simulink model "Controlador_com_Observador_Simulink(1)"  (R2019a)
settings: Solver=VariableStepAuto  StartTime=0.0  StopTime=10.0  RelTol=1e-3
values from neighbouring files (symbols this model uses):
  A = [0 1 0;0 0 1;-6 -11 -6]    [Projeto_controlador_observador(2).m]    (also in Q1_PCO(3).m = [0 1; -3 -4]; Q2_PCO(1).m = [0 1 0; 0 0 1; -12 -19 -8]; Q2_PCO(2).m = [0 1 0; 0 0 1; -12 -19 -8]; Q2_PCO(3).m = [0 1 0; 0 0 1; -12 -19 -8])
  B = [0 0 10]'    [Projeto_controlador_observador(2).m]    (also in Q1_PCO(3).m = [0 1]'; Q2_PCO(1).m = [0 0 1]'; Q2_PCO(2).m = [0 0 1]'; Q2_PCO(3).m = [0 0 1]')
  C = [1 0 0]    [Projeto_controlador_observador(2).m]    (also in Q1_PCO(3).m = [3 0]; Q2_PCO(1).m = [2 1 0]; Q2_PCO(2).m = [2 1 0]; Q2_PCO(3).m = [2 1 0])
  Kbar = acker(Abar,Bbar,polosMF)    [Projeto_controlador_observador(2).m]
  Ke = acker(A',C',autovaloresOBSV)'    [Projeto_controlador_observador(2).m]    (also in Q1_PCO(3).m = acker(A', C', autovaloresOBSV)'; Q2_PCO(1).m = acker(A', C', autovaloresOBSV)'; Q2_PCO(2).m = acker(A', C', autovaloresOBSV)'; Q2_PCO(3).m = acker(A', C', autovaloresOBSV)')
settings Model: Creator=rcard  LastModifiedBy=rcard

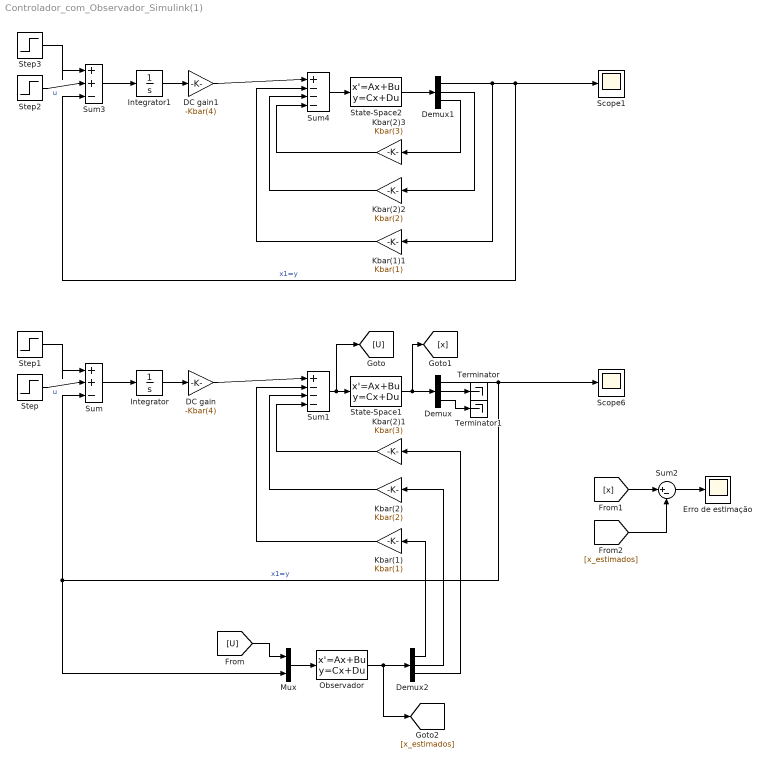
== system Controlador_com_Observador_Simulink(1) ==
  DC gain : Gain  Gain=-Kbar(4)
  DC gain1 : Gain  Gain=-Kbar(4)
  Demux : Demux  Outputs=3
  Demux1 : Demux  Outputs=3
  Demux2 : Demux  Outputs=3
  Erro de estimação : Scope
  Integrator : Integrator
  Integrator1 : Integrator
  Kbar(1) : Gain  Gain=Kbar(1)
  Kbar(1)1 : Gain  Gain=Kbar(1)
  Kbar(2) : Gain  Gain=Kbar(2)
  Kbar(2)1 : Gain  Gain=Kbar(3)
  Kbar(2)2 : Gain  Gain=Kbar(2)
  Kbar(2)3 : Gain  Gain=Kbar(3)
  Mux : Mux  Inputs=2
  Observador : StateSpace  A=(A-Ke*C)  B=[B Ke]  C=eye(3)  D=zeros(3,2)  InitialCondition=[1 -1 0.5]
  Scope1 : Scope
  Scope6 : Scope
  State-Space1 : StateSpace  A=A  B=B  C=eye(3)  D=zeros(3,1)  InitialCondition=[0 0 0]
  State-Space2 : StateSpace  A=A  B=B  C=eye(3)  D=zeros(3,1)  InitialCondition=[0 0 0]
  Step : Step  Time=5  SampleTime=0
  Step1 : Step  Time=0  SampleTime=1/20000
  Step2 : Step  Time=5  SampleTime=0
  Step3 : Step  Time=0  SampleTime=1/20000
  Sum : Sum  Inputs=|++-
  Sum1 : Sum  Inputs=|+---
  Sum2 : Sum  Inputs=|+-
  Sum3 : Sum  Inputs=|++-
  Sum4 : Sum  Inputs=|+---
  Terminator : Terminator
  Terminator1 : Terminator
  wires:
  Integrator/1 -> DC gain/1
  Sum/1 -> Integrator/1
  Kbar(1)/1 -> Sum1/2
  Kbar(2)/1 -> Sum1/3
  Sum1/1 -> [U], State-Space1/1
  DC gain/1 -> Sum1/1
  Demux/1 -> Mux/2, Sum/3, Scope6/1  "x1=y"
  State-Space1/1 -> [x], Demux/1
  Step1/1 -> Sum/1
  Kbar(2)1/1 -> Sum1/4
  Sum2/1 -> Erro de estimação/1
  Mux/1 -> Observador/1
  Step/1 -> Sum/2  "u"
  Observador/1 -> [x_estimados], Demux2/1
  Demux2/1 -> Kbar(1)/1
  Demux2/2 -> Kbar(2)/1
  Demux2/3 -> Kbar(2)1/1
  [U] -> Mux/1
  [x_estimados] -> Sum2/2
  [x] -> Sum2/1
  Kbar(2)3/1 -> Sum4/4
  Step3/1 -> Sum3/1
  Demux1/1 -> Kbar(1)1/1, Sum3/3, Scope1/1  "x1=y"
  State-Space2/1 -> Demux1/1
  DC gain1/1 -> Sum4/1
  Sum4/1 -> State-Space2/1
  Kbar(1)1/1 -> Sum4/2
  Kbar(2)2/1 -> Sum4/3
  Integrator1/1 -> DC gain1/1
  Sum3/1 -> Integrator1/1
  Step2/1 -> Sum3/2  "u"
  Demux1/3 -> Kbar(2)3/1
  Demux1/2 -> Kbar(2)2/1
  Demux/2 -> Terminator/1
  Demux/3 -> Terminator1/1
